simulink model "two_channel_wave_variable"  (R2019b)
settings: Solver=VariableStepAuto  StartTime=0.0  StopTime=20  FixedStep=0.001  MaxStep=0.2  RelTol=1e-3
libraries: simulink x2
settings Model: Creator=anuj  LastModifiedBy=manth
settings DebuggingCC: AlgebraicLoopMsg=none

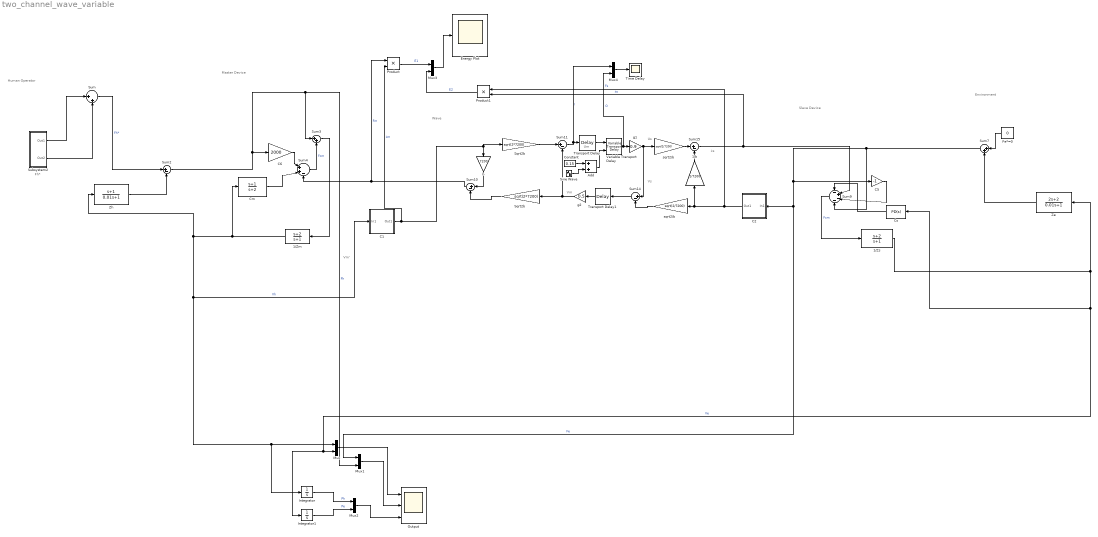
== system two_channel_wave_variable ==
  note: Wave
  note: ẋs
  note: Vs
  note: Us
  note: Vm
  note: Um
  note: Vm'
  note: Slave Device
  note: Environment
  note: Master Device
  note: Human Operator
  note: Fh*
  " Sqrt2b" : Gain  Gain=sqrt(2*7200)
  " sqrt2/b" : Gain  Gain=sqrt(2/7200)
  1/Zm : TransferFcn  Numerator=[1 2]  Denominator=[1 1]
  1/Zs : TransferFcn  Numerator=[1 2]  Denominator=[1 1]
  "1/b " : Gain  Gain=1/7200
  Add : Sum
  "C1 " : Subsystem
  "C2 " : Subsystem
  C5 : Gain  Gain=-1
  C6 : Gain  Gain=2000
  Cm : TransferFcn  Numerator=[1 1]  Denominator=[1 2]
  Constant : Constant  Value=0.15
  Cs : simulink/Continuous/PID Controller  Controller=PD  Form=Parallel  TimeDomain=Continuous-time  SampleTime=-1  IntegratorMethod=Forward Euler  FilterMethod=Forward Euler  ControllerParametersSource=internal  P=0.01  I=1  D=1  UseFilter=on  N=1000  TunerSelectOption=Transfer Function Based (PID Tuner App)  InitialConditionSource=internal  InitialConditionForIntegrator=0  InitialConditionForFilter=0  DifferentiatorICPrevScaledInput=0  ExternalReset=none  TrackingMode=off  Kt=1  LimitOutput=off  UpperSaturationLimit=inf  LowerSaturationLimit=-inf  LinearizeAsGain=on  AntiWindupMode=none  Kb=1  POutMin=[]  POutMax=[]  IOutMin=[]  IOutMax=[]  DOutMin=[]  DOutMax=[]  NOutMin=[]  NOutMax=[]  SumOutMin=[]  SumOutMax=[]  SaturationOutMin=[]  SaturationOutMax=[]  PParamMin=[]  PParamMax=[]  IParamMin=[]  IParamMax=[]  DParamMin=[]  DParamMax=[]  NParamMin=[]  NParamMax=[]  KbParamMin=[]  KbParamMax=[]  KtParamMin=[]  KtParamMax=[]  KbOutMin=[]  KbOutMax=[]  KtOutMin=[]  KtOutMax=[]  IntegratorOutMin=[]  IntegratorOutMax=[]  FilterOutMin=[]  FilterOutMax=[]  SumI1OutMin=[]  SumI1OutMax=[]  SumI2OutMin=[]  SumI2OutMax=[]  SumI3OutMin=[]  SumI3OutMax=[]  SumI4OutMin=[]  SumI4OutMax=[]  SumDOutMin=[]  SumDOutMax=[]  DifferentiatorOutMin=[]  DifferentiatorOutMax=[]  FilterDiffOutCoefMin=[]  FilterDiffOutCoefMax=[]  ReciprocalOutMin=[]  ReciprocalOutMax=[]  SumDenOutMin=[]  SumDenOutMax=[]  SumNumOutMin=[]  SumNumOutMax=[]  DivideOutMin=[]  DivideOutMax=[]  IntegratorContinuousStateAttributes=''  IntegratorStateMustResolveToSignalObject=off  IntegratorRTWStateStorageClass=Auto  FilterContinuousStateAttributes=''  FilterStateMustResolveToSignalObject=off  FilterRTWStateStorageClass=Auto  ParallelPVariant=InternalParameters  IdealPVariant=Disabled  IVariant=Disabled  DVariant=InternalParameters  IntegratorVariant=Disabled  SatVariant=Disabled  AWVariant=Disabled  PCopyVariant=Disabled  TRVariant=Disabled  FdbkBlocksVariant=Forward  IdealPFdbkVariant=Disabled  SatFdbkVariant=Disabled  DerivativeFilterVariant=ContFilter  NVariant=InternalParameters  NCopyVariant=Disabled  FilterICVariant=InternalICsFilter  IntegratorICVariant=Disabled  ExternalResetVariant=Disabled  TRSumVariant=Passthrough  SumFdbkVariant=Disabled  SumVariant=Sum_PD
  Energy Plot : Scope
  Fe*=0 : Constant  Value=0
  Integrator : Integrator
  Integrator1 : Integrator
  Mux{,1..4} (5 alike) : Mux  Inputs=2
  Output : Scope  NumInputPorts=3
  Product : Product
  Product1 : Product
  Sine Wave : Sin  Amplitude=0.1  Frequency=20  SampleTime=0
  Sqrt2b : Gain  Gain=sqrt(2*7200)
  Subsystem2 : Subsystem
  Sum : Sum  Inputs=|++
  Sum{2,10..11,14..15} (5 alike) : Sum  Inputs=|+-
  Sum3 : Sum  Inputs=|++
  Sum4 : Sum  Inputs=|++-
  Sum7 : Sum  Inputs=|++
  Sum9 : Sum  Inputs=-+--
  Time Delay : Scope
  Transport Delay : TransportDelay  DelayTime=0.15
  Transport Delay1 : TransportDelay  DelayTime=0.15
  Variable Transport Delay : VariableTransportDelay  VariableDelayType=Variable transport delay  MaximumDelay=10
  Ze : TransferFcn  Numerator=[2 2]  Denominator=[0.01 1]
  Zh : TransferFcn  Numerator=[1 1]  Denominator=[0.01 1]
  b : Gain  Gain=7200
  g1 : Gain  Gain=0.9
  g2 : Gain  Gain=0.5
  sqrt2/b : Gain  Gain=sqrt(2/7200)
  wires:
  Cm/1 -> Sum4/2
  Sum7/1 -> Mux1/1, "C2 "/1(In1), C5/1, Sum9/4  "Fe"
  1/Zm/1 -> Zh/1, "C1 "/1(In1), Integrator/1, Mux/1, Cm/1  "Vh"
  Cs/1 -> Sum9/1
  Fe*=0/1 -> Sum7/1
  Sum4/1 -> Sum3/2  "Fcm"
  1/Zs/1 -> Ze/1, Cs/1, Mux/2, Integrator1/1  "Ve"
  Sum9/1 -> 1/Zs/1  "Fcm"
  Sum3/1 -> 1/Zm/1
  Mux/1 -> Output/1
  Mux1/1 -> Output/2
  Ze/1 -> Sum7/2
  C6/1 -> Sum4/1
  C5/1 -> Sum9/3
  Sum2/1 -> Sum3/1, Mux1/2, C6/1  "Fh"
  Subsystem2/1(Out1) -> Sum/1
  Sum/1 -> Sum2/1  "Fh*"
  Subsystem2/2(Out2) -> Sum/2
  "C1 "/1(Out1) -> Product/2, b/1, " Sqrt2b"/1  "ẋm"
  Sqrt2b/1 -> Sum10/2
  "C2 "/1(Out1) -> Product1/1, "1/b "/1, " sqrt2/b"/1  "Fs"
  sqrt2/b/1 -> Sum15/1
  b/1 -> Sum10/1
  Sum10/1 -> Product/1, Sum4/3  "Fm"
  Sum14/1 -> Transport Delay1/1
  " Sqrt2b"/1 -> Sum11/1
  " sqrt2/b"/1 -> Sum14/2
  "1/b "/1 -> Sum15/2
  Sum15/1 -> Product1/2, Sum9/2  "ẋs"
  Integrator1/1 -> Mux2/2  "Pe"
  Integrator/1 -> Mux2/1  "Ph"
  Mux2/1 -> Output/3
  Zh/1 -> Sum2/2
  Mux3/1 -> Energy Plot/1
  Product/1 -> Mux3/1  "E1"
  Product1/1 -> Mux3/2  "E2"
  Transport Delay1/1 -> g2/1
  Variable Transport Delay/1 -> Mux4/2, g1/1  "O"
  Sum11/1 -> Transport Delay/1, Mux4/1  "I"
  Constant/1 -> Add/1
  Add/1 -> Variable Transport Delay/2
  Sine Wave/1 -> Add/2
  Mux4/1 -> Time Delay/1
  g1/1 -> Sum14/1, sqrt2/b/1
  g2/1 -> Sum11/2, Sqrt2b/1
  Transport Delay/1 -> Variable Transport Delay/1

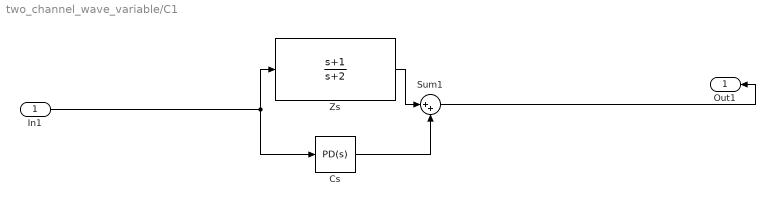
== system two_channel_wave_variable/C1  ==
  In1 : Inport
  Cs : simulink/Continuous/PID Controller  Controller=PD  Form=Parallel  TimeDomain=Continuous-time  SampleTime=-1  IntegratorMethod=Forward Euler  FilterMethod=Forward Euler  ControllerParametersSource=internal  P=0.01  I=1  D=1  UseFilter=on  N=1000  TunerSelectOption=Transfer Function Based (PID Tuner App)  InitialConditionSource=internal  InitialConditionForIntegrator=0  InitialConditionForFilter=0  DifferentiatorICPrevScaledInput=0  ExternalReset=none  TrackingMode=off  Kt=1  LimitOutput=off  UpperSaturationLimit=inf  LowerSaturationLimit=-inf  LinearizeAsGain=on  AntiWindupMode=none  Kb=1  POutMin=[]  POutMax=[]  IOutMin=[]  IOutMax=[]  DOutMin=[]  DOutMax=[]  NOutMin=[]  NOutMax=[]  SumOutMin=[]  SumOutMax=[]  SaturationOutMin=[]  SaturationOutMax=[]  PParamMin=[]  PParamMax=[]  IParamMin=[]  IParamMax=[]  DParamMin=[]  DParamMax=[]  NParamMin=[]  NParamMax=[]  KbParamMin=[]  KbParamMax=[]  KtParamMin=[]  KtParamMax=[]  KbOutMin=[]  KbOutMax=[]  KtOutMin=[]  KtOutMax=[]  IntegratorOutMin=[]  IntegratorOutMax=[]  FilterOutMin=[]  FilterOutMax=[]  SumI1OutMin=[]  SumI1OutMax=[]  SumI2OutMin=[]  SumI2OutMax=[]  SumI3OutMin=[]  SumI3OutMax=[]  SumI4OutMin=[]  SumI4OutMax=[]  SumDOutMin=[]  SumDOutMax=[]  DifferentiatorOutMin=[]  DifferentiatorOutMax=[]  FilterDiffOutCoefMin=[]  FilterDiffOutCoefMax=[]  ReciprocalOutMin=[]  ReciprocalOutMax=[]  SumDenOutMin=[]  SumDenOutMax=[]  SumNumOutMin=[]  SumNumOutMax=[]  DivideOutMin=[]  DivideOutMax=[]  IntegratorContinuousStateAttributes=''  IntegratorStateMustResolveToSignalObject=off  IntegratorRTWStateStorageClass=Auto  FilterContinuousStateAttributes=''  FilterStateMustResolveToSignalObject=off  FilterRTWStateStorageClass=Auto  ParallelPVariant=InternalParameters  IdealPVariant=Disabled  IVariant=Disabled  DVariant=InternalParameters  IntegratorVariant=Disabled  SatVariant=Disabled  AWVariant=Disabled  PCopyVariant=Disabled  TRVariant=Disabled  FdbkBlocksVariant=Forward  IdealPFdbkVariant=Disabled  SatFdbkVariant=Disabled  DerivativeFilterVariant=ContFilter  NVariant=InternalParameters  NCopyVariant=Disabled  FilterICVariant=InternalICsFilter  IntegratorICVariant=Disabled  ExternalResetVariant=Disabled  TRSumVariant=Passthrough  SumFdbkVariant=Disabled  SumVariant=Sum_PD
  Sum1 : Sum  Inputs=|++
  Zs : TransferFcn  Numerator=[1 1]  Denominator=[1 2]
  Out1 : Outport
  wires:
  In1/1 -> Cs/1, Zs/1
  Cs/1 -> Sum1/2
  Sum1/1 -> Out1/1
  Zs/1 -> Sum1/1

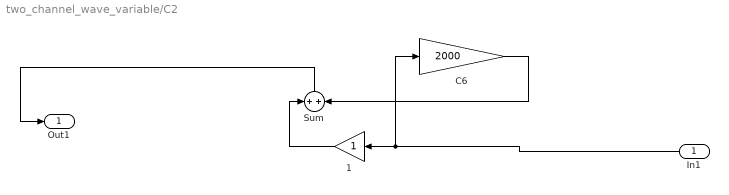
== system two_channel_wave_variable/C2  ==
  In1 : Inport
  1 : Gain
  C6 : Gain  Gain=2000
  Sum : Sum
  Out1 : Outport
  wires:
  C6/1 -> Sum/2
  In1/1 -> C6/1, 1/1
  1/1 -> Sum/1
  Sum/1 -> Out1/1

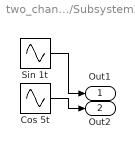
== system two_channel_wave_variable/Subsystem2 ==
  "Cos 5t " : Sin  Frequency=5  Phase=pi/2  SampleTime=0
  Sin 1t : Sin  SampleTime=0
  Out1 : Outport
  Out2 : Outport  Port=2
  wires:
  Sin 1t/1 -> Out1/1
  "Cos 5t "/1 -> Out2/1
